simulink library "hall_sensor_lib"  (R2021b)
settings: Solver=ode45  StartTime=0.0  StopTime=10.0  RelTol=1e-3
undefined symbols (not defined in the file or in its folder): SMO_params
libraries: simulink x3, $bdroot x2, tiiqmathlib x2, idelinklib_common x1
settings Model: Creator=The MathWorks, Inc.  LastModifiedBy=The MathWorks, Inc.
settings SolverCC: AlgebraicLoopSolver=TrustRegion
settings DataIOCC: LimitDataPoints=on  SaveFormat=Array  SignalLoggingSaveFormat=ModelDataLogs  ReturnWorkspaceOutputs=off
settings OptimizationCC: BlockReduction=off  BooleanDataType=off  ExpressionDepthLimit=2147483647  LifeSpan=inf
settings DebuggingCC: SaveWithParameterizedLinksMsg=none  UnderspecifiedInitializationDetection=Classic  MergeDetectMultiDrivingBlocksExec=none  SignalResolutionControl=TryResolveAllWithWarning  FcnCallInpInsideContextMsg=warning  StateNameClashWarn=warning  SFUnexpectedBacktrackingDiag=warning  SFNoUnconditionalDefaultTransitionDiag=warning  SFExecutionAtInitializationDiag=none  SFMachineParentedDataDiag=warning  ArithmeticOperatorsInVariantConditions=warning
settings HardwareCC: ProdBitPerPointer=32  ProdBitPerSizeT=32  ProdBitPerPtrDiffT=32  ProdLargestAtomicFloat=None  ProdIntDivRoundTo=Undefined  ProdEndianess=Unspecified  ProdWordSize=32  ProdHWDeviceType=32-bit Generic  TargetUnknown=on
settings ModelReferenceCC: PropagateSignalLabelsOutOfModel=off
settings SFSimCC: SimUseLocalCustomCode=off  CustomCodeUndefinedFunction=UseInterfaceOnly
settings RTWCC: RTWUseLocalCustomCode=off
settings CodeAppCC: StateflowObjectComments=on
settings GRTTargetCC: TargetLangStandard=C89/C90 (ANSI)  CombineOutputUpdateFcns=off  GRTInterface=on
settings ConfigComp: CovMetricSettings=dw  CovSaveCumulativeToWorkspaceVar=on  CovSaveSingleToWorkspaceVar=on  CovExternalEMLEnable=off  CovSFcnEnable=off

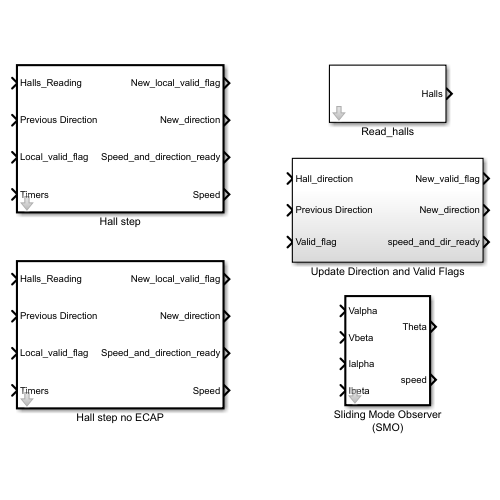
[thumbnail: Simulink's stored preview of the top-level diagram]
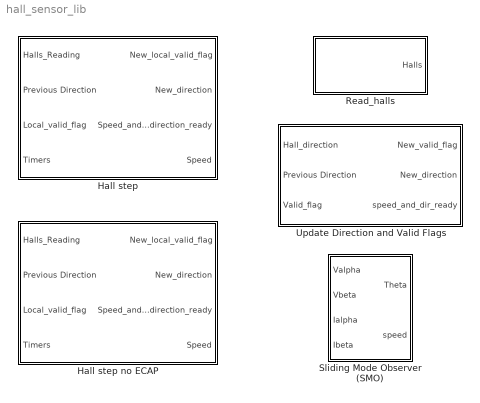
== system hall_sensor_lib ==
  Hall step : Subsystem  TreatAsAtomicUnit=on  mask(Hall decoder){hallRisingDir0=0, hallRisingDir1=0, hallFallingDir0=0, hallFallingDir1=0}
      mask prompts: hallRisingDir0 "Expected Halls reading after rising edge in direction 0"; hallRisingDir1 "Expected Halls reading after rising edge in direction 1"; hallFallingDir0 "Expected Halls reading after falling edge in direction 0"; hallFallingDir1 "Expected Halls reading after falling edge in direction 1"
      mask help:
      | This block updates speed, direction and valid flag signals depending on Hall sensor readings.
      | The inputs are:
      | - Halls reading.
      | - Current Direction
      | - Local valid flag.
      |
      | The outputs are:
      | - Local valid flag.
      | - Direction.
      | - Speed and direction valid flag.
  Hall step no ECAP : Subsystem  TreatAsAtomicUnit=on  mask(Hall decoder){hallRisingDir0=0, hallRisingDir1=0, hallFallingDir0=0, hallFallingDir1=0}
      mask prompts: hallRisingDir0 "Expected Halls reading after rising edge in direction 0"; hallRisingDir1 "Expected Halls reading after rising edge in direction 1"; hallFallingDir0 "Expected Halls reading after falling edge in direction 0"; hallFallingDir1 "Expected Halls reading after falling edge in direction 1"
      mask help:
      | This block updates speed, direction and valid flag signals depending on Hall sensor readings.
      | The inputs are:
      | - Halls reading.
      | - Current Direction
      | - Local valid flag.
      |
      | The outputs are:
      | - Local valid flag.
      | - Direction.
      | - Speed and direction valid flag.
  Read_halls : Subsystem  mask(Hall sensor reader){sample_time=-1}
      mask prompts: sample_time "Sample time:"
      mask help:
      | This block outputs the state of the 3 hall sensors placed on GPIO24, 25 and 26 of the F2808 DSP.
      |
      | 0 --> GPIO24 = 0, GPIO 25 = 0, GPIO 26 = 0
      | 1 --> GPIO24 = 1, GPIO 25 = 0, GPIO 26 = 0
      | 2 --> GPIO24 = 0, GPIO 25 = 1, GPIO 26 = 0
      | 3 --> GPIO24 = 1, GPIO 25 = 1, GPIO 26 = 0
      | 4 --> GPIO24 = 0, GPIO 25 = 0, GPIO 26 = 1
      | 5 --> GPIO24 = 1, GPIO 25 = 0, GPIO 26 = 1
      | 6 --> GPIO24 = 0, GPIO 25 = 1, GPIO 26 = 1
      | 7 --> GPIO24 = 1, GPIO 25 = 1, GPIO 26 = 1
  Sliding Mode Observer (SMO) : Subsystem  TreatAsAtomicUnit=on  mask(Sliding Mode Observer (SMO)){SMO_Kslide_gain=SMO_params.Kslide, SMO_Kslf_gain=SMO_params.Kslf, SMO_Fsmopos_gain=SMO_params.Fsmopos, SMO_Gsmopos_gain=SMO_params.Gsmopos, SMO_E0=SMO_params.E0, SMO_speed_loop_delay=SMO_params.Speed_loop_delay, SMO_speed_IIR_gain=SMO_params.Speed_IIR_filter_gain, Speed_PU_scaler=SMO_params.Speed_PU_scaler}
      mask prompts: SMO_Kslide_gain "Sliding gain"; SMO_Kslf_gain "Sliding filter gain"; SMO_Fsmopos_gain "Plant gain"; SMO_Gsmopos_gain "Control gain"; SMO_E0 "Internal saturation"; SMO_speed_loop_delay "Speed loop delay"; SMO_speed_IIR_gain "Speed IIR filter gain"; Speed_PU_scaler "Speed per unit scaler"
      mask help: Calculates position and speed using a Sliding Mode Observer algorithm.
      settings: MinAlgLoopOccurrences=on
      mask DialogControl ParameterGroupVar Prompt: SMO Parameters
  Update Direction and Valid Flags : Subsystem

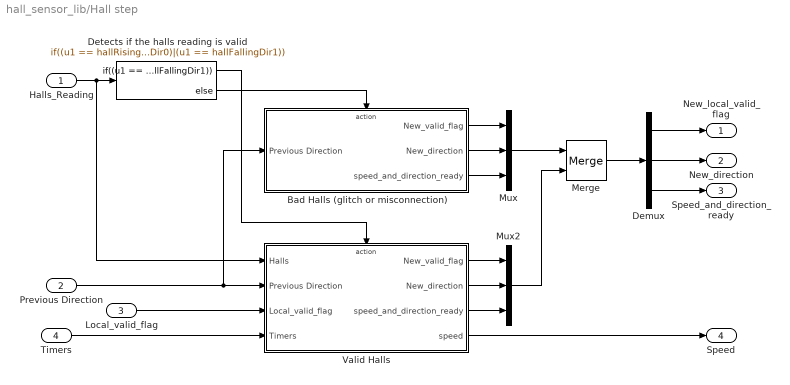
== system hall_sensor_lib/Hall step ==
  Halls_Reading : Inport
  Previous Direction : Inport  Port=2
  Local_valid_flag : Inport  Port=3
  Timers : Inport  Port=4
  Bad Halls (glitch or misconnection) : Subsystem  TreatAsAtomicUnit=on
  Demux : Demux  Outputs=3
  Detects if the halls reading is valid : If  IfExpression=(u1 == hallRisingDir0)|(u1 == hallRisingDir1)|(u1 == hallFallingDir0)|(u1 == hallFallingDir1)
  Merge : Merge
  Mux : Mux  Inputs=3
  Mux2 : Mux  Inputs=3
  Valid Halls : Subsystem  TreatAsAtomicUnit=on
  New_local_valid_flag : Outport
  New_direction : Outport  Port=2
  Speed_and_direction_ready : Outport  Port=3
  Speed : Outport  Port=4
  wires:
  Detects if the halls reading is valid/1 -> Valid Halls/Action
  Halls_Reading/1 -> Detects if the halls reading is valid/1, Valid Halls/1(Halls)
  Previous Direction/1 -> Bad Halls (glitch or misconnection)/1(Previous Direction), Valid Halls/2(Previous Direction)
  Bad Halls (glitch or misconnection)/1(New_valid_flag) -> Mux/1
  Bad Halls (glitch or misconnection)/2(New_direction) -> Mux/2
  Valid Halls/1(New_valid_flag) -> Mux2/1
  Valid Halls/2(New_direction) -> Mux2/2
  Valid Halls/3(speed_and_direction_ready) -> Mux2/3
  Bad Halls (glitch or misconnection)/3(speed_and_direction_ready) -> Mux/3
  Merge/1 -> Demux/1
  Detects if the halls reading is valid/2 -> Bad Halls (glitch or misconnection)/Action
  Mux/1 -> Merge/1
  Mux2/1 -> Merge/2
  Demux/1 -> New_local_valid_flag/1
  Demux/3 -> Speed_and_direction_ready/1
  Demux/2 -> New_direction/1
  Local_valid_flag/1 -> Valid Halls/3(Local_valid_flag)
  Timers/1 -> Valid Halls/4(Timers)
  Valid Halls/4(speed) -> Speed/1

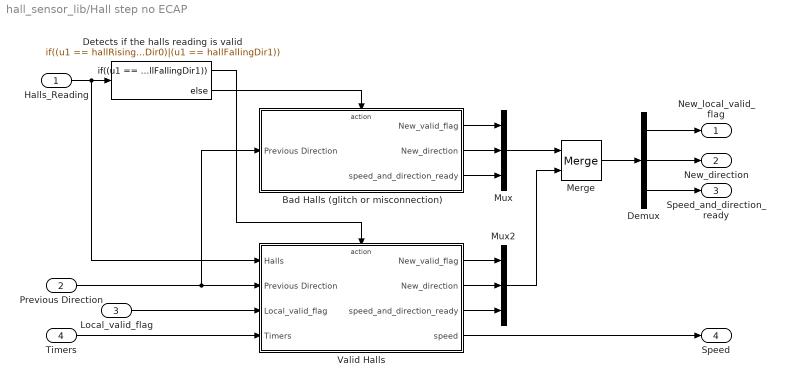
== system hall_sensor_lib/Hall step no ECAP ==
  Halls_Reading : Inport
  Previous Direction : Inport  Port=2
  Local_valid_flag : Inport  Port=3
  Timers : Inport  Port=4
  Bad Halls (glitch or misconnection) : Subsystem  TreatAsAtomicUnit=on
  Demux : Demux  Outputs=3
  Detects if the halls reading is valid : If  IfExpression=(u1 == hallRisingDir0)|(u1 == hallRisingDir1)|(u1 == hallFallingDir0)|(u1 == hallFallingDir1)
  Merge : Merge
  Mux : Mux  Inputs=3
  Mux2 : Mux  Inputs=3
  Valid Halls : Subsystem  TreatAsAtomicUnit=on
  New_local_valid_flag : Outport
  New_direction : Outport  Port=2
  Speed_and_direction_ready : Outport  Port=3
  Speed : Outport  Port=4
  wires:
  Valid Halls/4(speed) -> Speed/1
  Timers/1 -> Valid Halls/4(Timers)
  Local_valid_flag/1 -> Valid Halls/3(Local_valid_flag)
  Demux/2 -> New_direction/1
  Demux/3 -> Speed_and_direction_ready/1
  Demux/1 -> New_local_valid_flag/1
  Mux2/1 -> Merge/2
  Mux/1 -> Merge/1
  Detects if the halls reading is valid/2 -> Bad Halls (glitch or misconnection)/Action
  Merge/1 -> Demux/1
  Bad Halls (glitch or misconnection)/3(speed_and_direction_ready) -> Mux/3
  Valid Halls/3(speed_and_direction_ready) -> Mux2/3
  Valid Halls/2(New_direction) -> Mux2/2
  Valid Halls/1(New_valid_flag) -> Mux2/1
  Bad Halls (glitch or misconnection)/2(New_direction) -> Mux/2
  Bad Halls (glitch or misconnection)/1(New_valid_flag) -> Mux/1
  Previous Direction/1 -> Valid Halls/2(Previous Direction), Bad Halls (glitch or misconnection)/1(Previous Direction)
  Halls_Reading/1 -> Valid Halls/1(Halls), Detects if the halls reading is valid/1
  Detects if the halls reading is valid/1 -> Valid Halls/Action

== system hall_sensor_lib/Read_halls ==
  Bitwise Operator : simulink/Logic and Bit Operations/Bitwise Operator  logicop=AND  UseBitMask=on  BitMask=hex2dec('07000000')  BitMaskRealWorld=Stored Integer
  Data Type Conversion : DataTypeConversion  OutDataTypeStr=uint16  ConvertRealWorld=Stored Integer (SI)
  Read GPIO DAT register : idelinklib_common/Memory Copy  copyFrom=Specified source code symbol  copyFromAddressSource=Specify via dialog  copyFromAddress=hex2dec('6FC1')  copyFromSrcCode=&GpioDataRegs.GPADAT.all  dataTypeFrom=uint32  dataDimensionFrom=1  useOffsetFrom=off  offsetFromSrc=Specify via dialog  offsetFrom=0  strideFrom=1  copyTo=Output port  copyToAddressSource=Specify via dialog  copyToAddress=hex2dec('00002000')  copyToSrcCode=GpioDataRegs.GPADAT.bit.GPIO24  dataTypeTo=uint32  useOffsetTo=off  offsetToSrc=Specify via dialog  offsetTo=0  strideTo=1  sampleTime=-1  useInitValue=off  initValueSrc=Specify constant value  initValue=1  initValueSrcCode=myInitValueVariable  useAsMask=off  maskOperator=bitwise AND  useTermValue=off  termValue=1  isRealtimeEnabled=off  emitCCBeforeWrite=off  CCBeforeWrite=/* Custom Code Before Write*/  emitCCAfterWrite=off  CCAfterWrite=/* Custom Code After Write*/  useDMACopy=off  enableBlockingMode=off
      settings: SourceProductBaseCode=ME
  Shift Arithmetic : ArithShift  BitShiftNumber=24
  Halls : Outport
  wires:
  Shift Arithmetic/1 -> Data Type Conversion/1
  Read GPIO DAT register/1 -> Bitwise Operator/1
  Bitwise Operator/1 -> Shift Arithmetic/1
  Data Type Conversion/1 -> Halls/1

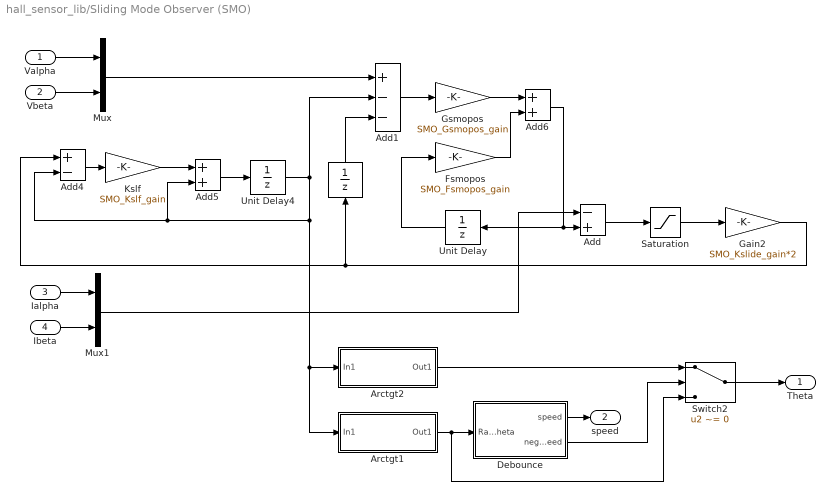
== system hall_sensor_lib/Sliding Mode Observer (SMO) ==
  Valpha : Inport
  Vbeta : Inport  Port=2
  Ialpha : Inport  Port=3
  Ibeta : Inport  Port=4
  " " : UnitDelay  SampleTime=-1  HasFrameUpgradeWarning=on
  Add : Sum  Inputs=-+  OutDataTypeStr=Inherit: Same as first input
  Add1 : Sum  Inputs=+--  OutDataTypeStr=Inherit: Inherit via back propagation
  Add4 : Sum  Inputs=+-  OutDataTypeStr=Inherit: Same as first input
  Add5 : Sum  OutDataTypeStr=Inherit: Same as first input
  Add6 : Sum  OutDataTypeStr=Inherit: Same as first input
  Arctgt1 : Subsystem
  Arctgt2 : Subsystem
  Debounce : Subsystem
  Fsmopos : Gain  Gain=SMO_Fsmopos_gain  OutDataTypeStr=Inherit: Same as input  ParamDataTypeStr=Inherit: Same as input
  Gain2 : Gain  Gain=SMO_Kslide_gain*2  OutDataTypeStr=Inherit: Same as input  ParamDataTypeStr=Inherit: Same as input
  Gsmopos : Gain  Gain=SMO_Gsmopos_gain  OutDataTypeStr=Inherit: Same as input  ParamDataTypeStr=Inherit: Same as input
  Kslf : Gain  Gain=SMO_Kslf_gain  OutDataTypeStr=Inherit: Same as input  ParamDataTypeStr=Inherit: Same as input
  Mux : Mux  Inputs=2
  Mux1 : Mux  Inputs=2
  Saturation : Saturate  UpperLimit=SMO_E0  LowerLimit=-SMO_E0
  Switch2 : Switch  Criteria=u2 ~= 0
  Unit Delay : UnitDelay  SampleTime=-1  HasFrameUpgradeWarning=on
  Unit Delay4 : UnitDelay  SampleTime=-1  HasFrameUpgradeWarning=on
  Theta : Outport
  speed : Outport  Port=2
  wires:
  Unit Delay/1 -> Fsmopos/1
  " "/1 -> Add1/3
  Add1/1 -> Gsmopos/1
  Valpha/1 -> Mux/1
  Vbeta/1 -> Mux/2
  Mux/1 -> Add1/1
  Add4/1 -> Kslf/1
  Unit Delay4/1 -> Arctgt2/1(In1), Arctgt1/1(In1), Add5/2, Add4/2, Add1/2
  Kslf/1 -> Add5/1
  Add5/1 -> Unit Delay4/1
  Gsmopos/1 -> Add6/1
  Fsmopos/1 -> Add6/2
  Add6/1 -> Add/2, Unit Delay/1
  Ialpha/1 -> Mux1/1
  Ibeta/1 -> Mux1/2
  Gain2/1 -> " "/1, Add4/1
  Mux1/1 -> Add/1
  Arctgt1/1(Out1) -> Debounce/1(Raw_theta), Switch2/3
  Arctgt2/1(Out1) -> Switch2/1
  Switch2/1 -> Theta/1
  Debounce/1(speed) -> speed/1
  Debounce/2(negative speed) -> Switch2/2
  Saturation/1 -> Gain2/1
  Add/1 -> Saturation/1

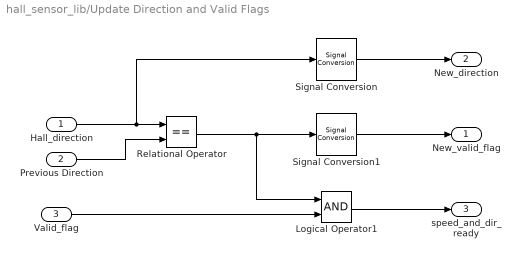
== system hall_sensor_lib/Update Direction and Valid Flags ==
  Hall_direction : Inport
  Previous Direction : Inport  Port=2
  Valid_flag : Inport  Port=3
  Logical Operator1 : Logic  AllPortsSameDT=off  OutDataTypeStr=uint(16)
  Relational Operator : RelationalOperator  Operator===  OutDataTypeStr=uint(16)  RndMeth=Nearest
  Signal Conversion : SignalConversion  OverrideOpt=on
  Signal Conversion1 : SignalConversion  OverrideOpt=on
  New_valid_flag : Outport
  New_direction : Outport  Port=2
  speed_and_dir_ready : Outport  Port=3
  wires:
  Previous Direction/1 -> Relational Operator/2
  Hall_direction/1 -> Relational Operator/1, Signal Conversion/1
  Valid_flag/1 -> Logical Operator1/2
  Relational Operator/1 -> Signal Conversion1/1, Logical Operator1/1
  Signal Conversion/1 -> New_direction/1
  Logical Operator1/1 -> speed_and_dir_ready/1
  Signal Conversion1/1 -> New_valid_flag/1

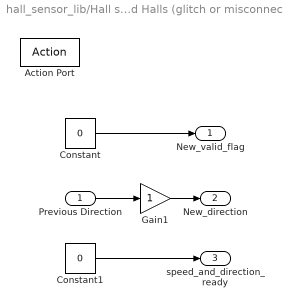
== system hall_sensor_lib/Hall step/Bad Halls (glitch or misconnection) ==
  Previous Direction : Inport
  Action Port : ActionPort
  Constant : Constant  Value=0  OutDataTypeStr=uint16
  Constant1 : Constant  Value=0  OutDataTypeStr=uint16
  Gain1 : Gain  OutDataTypeStr=Inherit: Same as input  ParamDataTypeStr=Inherit: Same as input
  New_valid_flag : Outport
  New_direction : Outport  Port=2
  speed_and_direction_ready : Outport  Port=3
  wires:
  Gain1/1 -> New_direction/1
  Previous Direction/1 -> Gain1/1
  Constant/1 -> New_valid_flag/1
  Constant1/1 -> speed_and_direction_ready/1

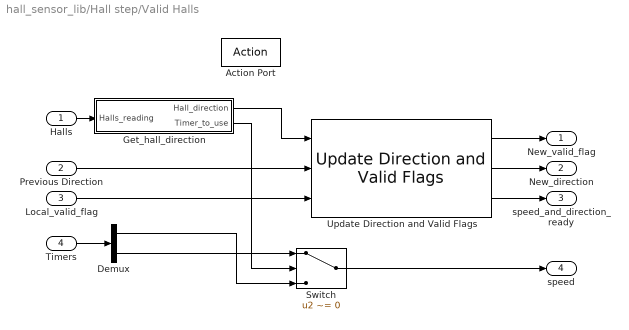
== system hall_sensor_lib/Hall step/Valid Halls ==
  Halls : Inport
  Previous Direction : Inport  Port=2
  Local_valid_flag : Inport  Port=3
  Timers : Inport  Port=4
  Action Port : ActionPort
  Demux : Demux  Outputs=2
  Get_hall_direction : Subsystem
  Switch : Switch  Criteria=u2 ~= 0
  Update Direction and Valid Flags : $bdroot/Update Direction and Valid Flags  SystemSampleTime=-1  VariantActivationTime=update diagram  Latency=0  AutoFrameSizeCalculation=off
  New_valid_flag : Outport
  New_direction : Outport  Port=2
  speed_and_direction_ready : Outport  Port=3
  speed : Outport  Port=4
  wires:
  Get_hall_direction/1(Hall_direction) -> Update Direction and Valid Flags/1
  Previous Direction/1 -> Update Direction and Valid Flags/2
  Local_valid_flag/1 -> Update Direction and Valid Flags/3
  Update Direction and Valid Flags/1 -> New_valid_flag/1
  Update Direction and Valid Flags/2 -> New_direction/1
  Update Direction and Valid Flags/3 -> speed_and_direction_ready/1
  Halls/1 -> Get_hall_direction/1(Halls_reading)
  Switch/1 -> speed/1
  Timers/1 -> Demux/1
  Get_hall_direction/2(Timer_to_use) -> Switch/2
  Demux/2 -> Switch/1
  Demux/1 -> Switch/3

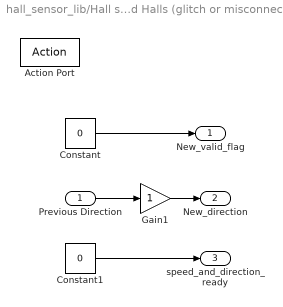
== system hall_sensor_lib/Hall step no ECAP/Bad Halls (glitch or misconnection) ==
  Previous Direction : Inport
  Action Port : ActionPort
  Constant : Constant  Value=0  OutDataTypeStr=uint16
  Constant1 : Constant  Value=0  OutDataTypeStr=uint16
  Gain1 : Gain  OutDataTypeStr=Inherit: Same as input  ParamDataTypeStr=Inherit: Same as input
  New_valid_flag : Outport
  New_direction : Outport  Port=2
  speed_and_direction_ready : Outport  Port=3
  wires:
  Constant1/1 -> speed_and_direction_ready/1
  Constant/1 -> New_valid_flag/1
  Previous Direction/1 -> Gain1/1
  Gain1/1 -> New_direction/1

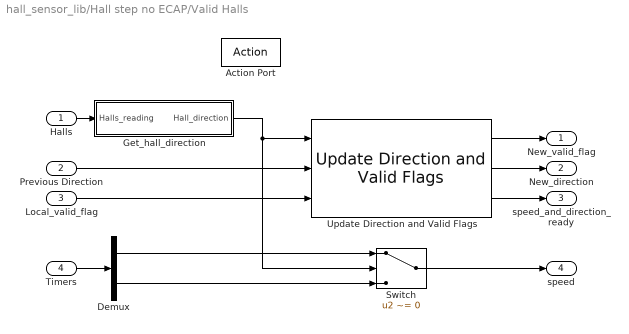
== system hall_sensor_lib/Hall step no ECAP/Valid Halls ==
  Halls : Inport
  Previous Direction : Inport  Port=2
  Local_valid_flag : Inport  Port=3
  Timers : Inport  Port=4
  Action Port : ActionPort
  Demux : Demux  Outputs=2
  Get_hall_direction : Subsystem
  Switch : Switch  Criteria=u2 ~= 0
  Update Direction and Valid Flags : $bdroot/Update Direction and Valid Flags  SystemSampleTime=-1  VariantActivationTime=update diagram  Latency=0  AutoFrameSizeCalculation=off
  New_valid_flag : Outport
  New_direction : Outport  Port=2
  speed_and_direction_ready : Outport  Port=3
  speed : Outport  Port=4
  wires:
  Get_hall_direction/1(Hall_direction) -> Update Direction and Valid Flags/1, Switch/2
  Timers/1 -> Demux/1
  Switch/1 -> speed/1
  Halls/1 -> Get_hall_direction/1(Halls_reading)
  Update Direction and Valid Flags/3 -> speed_and_direction_ready/1
  Update Direction and Valid Flags/2 -> New_direction/1
  Update Direction and Valid Flags/1 -> New_valid_flag/1
  Local_valid_flag/1 -> Update Direction and Valid Flags/3
  Previous Direction/1 -> Update Direction and Valid Flags/2
  Demux/1 -> Switch/1
  Demux/2 -> Switch/3

== system hall_sensor_lib/Sliding Mode Observer (SMO)/Arctgt1 ==
  In1 : Inport
  Arctangent IQN : tiiqmathlib/Arctangent IQN  tanOption=atan2PU (per unit)
      settings: SourceProductBaseCode=TIC2000
  Demux1 : Demux  Outputs=2
  Gain1 : Gain  Gain=-1  OutDataTypeStr=Inherit: Same as input  ParamDataTypeStr=Inherit: Same as input
  Out1 : Outport
  wires:
  In1/1 -> Demux1/1
  Arctangent IQN/1 -> Out1/1
  Demux1/1 -> Gain1/1
  Gain1/1 -> Arctangent IQN/2
  Demux1/2 -> Arctangent IQN/1

== system hall_sensor_lib/Sliding Mode Observer (SMO)/Arctgt2 ==
  In1 : Inport
  Arctangent IQN : tiiqmathlib/Arctangent IQN  tanOption=atan2PU (per unit)
      settings: SourceProductBaseCode=TIC2000
  Demux1 : Demux  Outputs=2
  Gain1 : Gain  Gain=-1  OutDataTypeStr=Inherit: Same as input  ParamDataTypeStr=Inherit: Same as input
  Out1 : Outport
  wires:
  In1/1 -> Demux1/1
  Arctangent IQN/1 -> Out1/1
  Demux1/1 -> Arctangent IQN/2
  Demux1/2 -> Gain1/1
  Gain1/1 -> Arctangent IQN/1

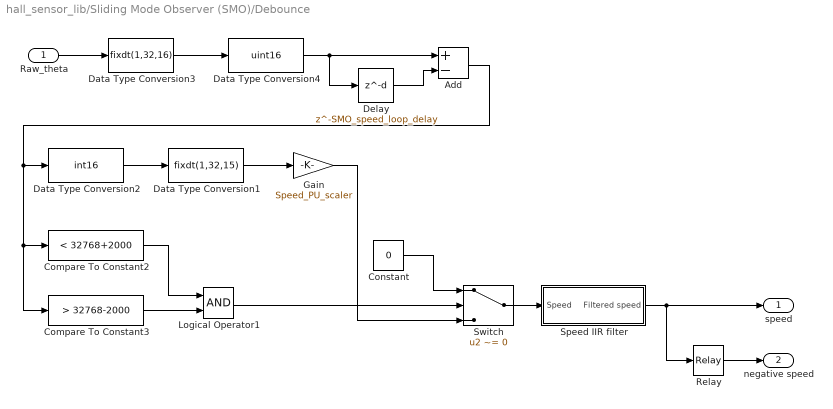
== system hall_sensor_lib/Sliding Mode Observer (SMO)/Debounce ==
  Raw_theta : Inport
  Add : Sum  Inputs=+-  OutDataTypeStr=uint16
  Compare To Constant2 : simulink/Logic and Bit Operations/Compare To Constant  relop=<  const=32768+2000  OutDataTypeStr=boolean
  Compare To Constant3 : simulink/Logic and Bit Operations/Compare To Constant  relop=>  const=32768-2000  OutDataTypeStr=boolean
  Constant : Constant  Value=0  OutDataTypeStr=fixdt(1,32,17)
  Data Type Conversion1 : DataTypeConversion  OutDataTypeStr=fixdt(1,32,15)  ConvertRealWorld=Stored Integer (SI)
  Data Type Conversion2 : DataTypeConversion  OutDataTypeStr=int16  ConvertRealWorld=Stored Integer (SI)
  Data Type Conversion3 : DataTypeConversion  OutDataTypeStr=fixdt(1,32,16)
  Data Type Conversion4 : DataTypeConversion  OutDataTypeStr=uint16  ConvertRealWorld=Stored Integer (SI)
  Delay : Delay  DelayLength=SMO_speed_loop_delay
  Gain : Gain  Gain=Speed_PU_scaler  ParamDataTypeStr=fixdt(1,32,17)  OutDataTypeStr=fixdt(1,32,17)
  Logical Operator1 : Logic  AllPortsSameDT=off  OutDataTypeStr=boolean
  Relay : Relay  OnSwitchValue=0.05  OffSwitchValue=-0.05  OnOutputValue=0  OffOutputValue=1
  Speed IIR filter : Subsystem
  Switch : Switch  Criteria=u2 ~= 0
  speed : Outport
  negative speed : Outport  Port=2
  wires:
  Add/1 -> Compare To Constant3/1, Compare To Constant2/1, Data Type Conversion2/1
  Raw_theta/1 -> Data Type Conversion3/1
  Delay/1 -> Add/2
  Data Type Conversion2/1 -> Data Type Conversion1/1
  Data Type Conversion3/1 -> Data Type Conversion4/1
  Data Type Conversion1/1 -> Gain/1
  Data Type Conversion4/1 -> Add/1, Delay/1
  Compare To Constant2/1 -> Logical Operator1/1
  Compare To Constant3/1 -> Logical Operator1/2
  Logical Operator1/1 -> Switch/2
  Constant/1 -> Switch/1
  Switch/1 -> Speed IIR filter/1(Speed)
  Gain/1 -> Switch/3
  Relay/1 -> negative speed/1
  Speed IIR filter/1(Filtered speed) -> speed/1, Relay/1

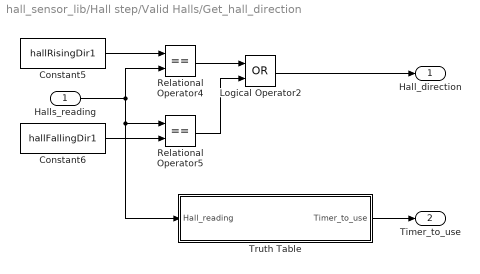
== system hall_sensor_lib/Hall step/Valid Halls/Get_hall_direction ==
  Halls_reading : Inport
  Constant5 : Constant  Value=hallRisingDir1  OutDataTypeStr=uint16
  Constant6 : Constant  Value=hallFallingDir1  OutDataTypeStr=uint16
  Logical Operator2 : Logic  Operator=OR  AllPortsSameDT=off  OutDataTypeStr=uint(16)
  Relational Operator4 : RelationalOperator  Operator===  OutDataTypeStr=uint(16)  RndMeth=Nearest
  Relational Operator5 : RelationalOperator  Operator===  OutDataTypeStr=uint(16)  RndMeth=Nearest
  Truth Table : Truth Table  TreatAsAtomicUnit=on
  Hall_direction : Outport
  Timer_to_use : Outport  Port=2
  wires:
  Constant6/1 -> Relational Operator5/2
  Constant5/1 -> Relational Operator4/1
  Relational Operator5/1 -> Logical Operator2/2
  Relational Operator4/1 -> Logical Operator2/1
  Halls_reading/1 -> Relational Operator4/2, Relational Operator5/1, Truth Table/1(Hall_reading)
  Logical Operator2/1 -> Hall_direction/1
  Truth Table/1(Timer_to_use) -> Timer_to_use/1

== system hall_sensor_lib/Hall step no ECAP/Valid Halls/Get_hall_direction ==
  Halls_reading : Inport
  Constant5 : Constant  Value=hallRisingDir1  OutDataTypeStr=uint16
  Constant6 : Constant  Value=hallFallingDir1  OutDataTypeStr=uint16
  Logical Operator2 : Logic  Operator=OR  AllPortsSameDT=off  OutDataTypeStr=uint(16)
  Relational Operator4 : RelationalOperator  Operator===  OutDataTypeStr=uint(16)  RndMeth=Nearest
  Relational Operator5 : RelationalOperator  Operator===  OutDataTypeStr=uint(16)  RndMeth=Nearest
  Hall_direction : Outport
  wires:
  Logical Operator2/1 -> Hall_direction/1
  Halls_reading/1 -> Relational Operator5/1, Relational Operator4/2
  Relational Operator4/1 -> Logical Operator2/1
  Relational Operator5/1 -> Logical Operator2/2
  Constant5/1 -> Relational Operator4/1
  Constant6/1 -> Relational Operator5/2

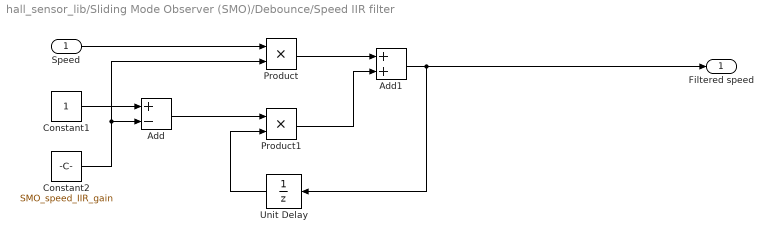
== system hall_sensor_lib/Sliding Mode Observer (SMO)/Debounce/Speed IIR filter ==
  Speed : Inport
  Add : Sum  Inputs=+-
  Add1 : Sum
  Constant1 : Constant  OutDataTypeStr=fixdt(1,32,17)
  Constant2 : Constant  Value=SMO_speed_IIR_gain  OutDataTypeStr=fixdt(1,32,17)
  Product : Product  OutDataTypeStr=Inherit: Same as first input
  Product1 : Product  OutDataTypeStr=Inherit: Same as first input
  Unit Delay : UnitDelay  SampleTime=-1  HasFrameUpgradeWarning=on
  Filtered speed : Outport
  wires:
  Speed/1 -> Product/1
  Add1/1 -> Unit Delay/1, Filtered speed/1
  Constant1/1 -> Add/1
  Constant2/1 -> Product/2, Add/2
  Product/1 -> Add1/1
  Add/1 -> Product1/1
  Unit Delay/1 -> Product1/2
  Product1/1 -> Add1/2

== matlab function hall_sensor_lib/Hall step/Valid Halls/Get_hall_direction/Truth Table ==
  data: Hall_reading input; Timer_to_use output uint16; hallRisingDir1 parameter uint16; hallRisingDir0 parameter uint16; hallFallingDir0 parameter uint16; hallFallingDir1 parameter uint16
function Timer_to_use = fcn(Hall_reading, hallRisingDir1, hallRisingDir0, hallFallingDir0, hallFallingDir1)

aVarTruthTableCondition_1 = false;
aVarTruthTableCondition_2 = false;



aVarTruthTableCondition_1 = logical((Hall_reading == hallFallingDir0) || (Hall_reading == hallFallingDir1));


aVarTruthTableCondition_2 = logical((Hall_reading == hallRisingDir0) || (Hall_reading == hallRisingDir1));

if (aVarTruthTableCondition_1)
    aFcnTruthTableAction_2();
else % Default
    aFcnTruthTableAction_1();
end

function aFcnTruthTableAction_1()

% Example action 1 called from D1 & D2 column in condition table

Timer_to_use = uint16(0);

function aFcnTruthTableAction_2()

% Example action 2 called from D3 column in condition table

Timer_to_use = uint16(1);
